simulink model "space_shuttle"  (R2020a)
settings: Solver=ode45  StartTime=0.0  StopTime=8  FixedStep=ts  MaxStep=tpwm/100  RelTol=1e-3
values from neighbouring files (symbols this model uses):
  alphac0 = 0.30    (= 0.3)    [main.m]
  alphac1 = 0.27    [main.m]
  alphanom = 0.3    [main.m]
  E = 0.05    [main.m]
  Kd = 0.75    [main.m]
  Ki = 2.70    (= 2.7)    [main.m]
  Kp = 1.25    [main.m]
  tpwm = 0.02    [main.m]
  ts = 0.1    [main.m]
  tstep = 1    [equarec.m]    (also in main.m; navettecontinue.m)
  u0 = 0    [main.m]
  u1 = 0.05    [main.m]
  x0 = [0;0]    [main.m]    (also in ore.m = x0(:))
undefined symbols (not defined in the file or in its folder): denctf, dendtf, DiscIntNeverNeededParam, numctf, numdtf
libraries: simulink x4
settings Model: Creator=albanfelix  LastModifiedBy=albanfelix

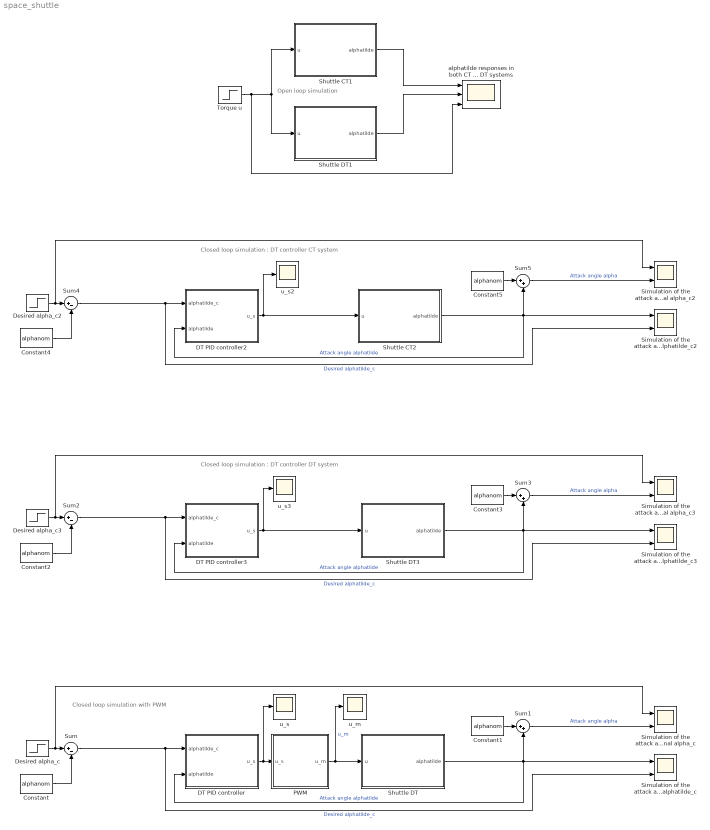
== system space_shuttle ==
  note: Open loop simulation
  note: Closed loop simulation with PWM
  note: Closed loop simulation : DT controller DT system
  note: Closed loop simulation : DT controller CT system
  Constant{,1..5} (6 alike) : Constant  Value=alphanom  SampleTime=ts
  DT PID controller : Subsystem
  DT PID controller2 : Subsystem
  DT PID controller3 : Subsystem
  Desired alpha_c : Step  Time=tstep  Before=alphac0  After=alphac1  SampleTime=ts
  Desired alpha_c2 : Step  Time=tstep  Before=alphac0  After=alphac1  SampleTime=ts
  Desired alpha_c3 : Step  Time=tstep  Before=alphac0  After=alphac1  SampleTime=ts
  PWM : Subsystem
  Shuttle CT1 : Subsystem
  Shuttle CT2 : Subsystem
  Shuttle DT : Subsystem
  Shuttle DT1 : Subsystem
  Shuttle DT3 : Subsystem
  Simulation of the attack angle alpha in function of the desired signal alpha_c : Scope  NumInputPorts=2
  Simulation of the attack angle alpha in function of the desired signal alpha_c2 : Scope  NumInputPorts=2
  Simulation of the attack angle alpha in function of the desired signal alpha_c3 : Scope  NumInputPorts=2
  Simulation of the attack angle alphatilde in function of the desired signal alphatilde_c : Scope  NumInputPorts=2
  Simulation of the attack angle alphatilde in function of the desired signal alphatilde_c2 : Scope  NumInputPorts=2
  Simulation of the attack angle alphatilde in function of the desired signal alphatilde_c3 : Scope  NumInputPorts=2
  Sum : Sum  Inputs=|+-
  Sum1 : Sum  Inputs=|++
  Sum2 : Sum  Inputs=|+-
  Sum3 : Sum  Inputs=|++
  Sum4 : Sum  Inputs=|+-
  Sum5 : Sum  Inputs=|++
  Torque u : Step  Time=tstep  Before=u0  After=u1  SampleTime=ts
  alphatilde responses in both CT and DT systems : Scope  NumInputPorts=3
  u_m : Scope
  u_s : Scope
  u_s2 : Scope
  u_s3 : Scope
  wires:
  Shuttle DT1/1(alphatilde) -> alphatilde responses in both CT and DT systems/2
  Shuttle DT/1(alphatilde) -> Simulation of the attack angle alphatilde in function of the desired signal alphatilde_c/1, DT PID controller/2(alphatilde), Sum1/2  "Attack angle alphatilde"
  DT PID controller/1(u_s) -> u_s/1, PWM/1(u_s)
  PWM/1(u_m) -> Shuttle DT/1(u), u_m/1  "u_m"
  Shuttle CT1/1(alphatilde) -> alphatilde responses in both CT and DT systems/1
  Sum/1 -> Simulation of the attack angle alphatilde in function of the desired signal alphatilde_c/2, DT PID controller/1(alphatilde_c)  "Desired alphatilde_c"
  Desired alpha_c/1 -> Simulation of the attack angle alpha in function of the desired signal alpha_c/1, Sum/1
  Constant/1 -> Sum/2
  Constant1/1 -> Sum1/1
  Sum1/1 -> Simulation of the attack angle alpha in function of the desired signal alpha_c/2  "Attack angle alpha"
  DT PID controller3/1(u_s) -> u_s3/1, Shuttle DT3/1(u)
  Sum3/1 -> Simulation of the attack angle alpha in function of the desired signal alpha_c3/2  "Attack angle alpha"
  Shuttle DT3/1(alphatilde) -> Simulation of the attack angle alphatilde in function of the desired signal alphatilde_c3/1, DT PID controller3/2(alphatilde), Sum3/2  "Attack angle alphatilde"
  Sum2/1 -> Simulation of the attack angle alphatilde in function of the desired signal alphatilde_c3/2, DT PID controller3/1(alphatilde_c)  "Desired alphatilde_c"
  Desired alpha_c3/1 -> Simulation of the attack angle alpha in function of the desired signal alpha_c3/1, Sum2/1
  Constant2/1 -> Sum2/2
  Constant3/1 -> Sum3/1
  Sum5/1 -> Simulation of the attack angle alpha in function of the desired signal alpha_c2/2  "Attack angle alpha"
  Constant5/1 -> Sum5/1
  Constant4/1 -> Sum4/2
  Desired alpha_c2/1 -> Simulation of the attack angle alpha in function of the desired signal alpha_c2/1, Sum4/1
  DT PID controller2/1(u_s) -> Shuttle CT2/1(u), u_s2/1
  Shuttle CT2/1(alphatilde) -> Simulation of the attack angle alphatilde in function of the desired signal alphatilde_c2/1, DT PID controller2/2(alphatilde), Sum5/2  "Attack angle alphatilde"
  Sum4/1 -> Simulation of the attack angle alphatilde in function of the desired signal alphatilde_c2/2, DT PID controller2/1(alphatilde_c)  "Desired alphatilde_c"
  Torque u/1 -> alphatilde responses in both CT and DT systems/3, Shuttle CT1/1(u), Shuttle DT1/1(u)

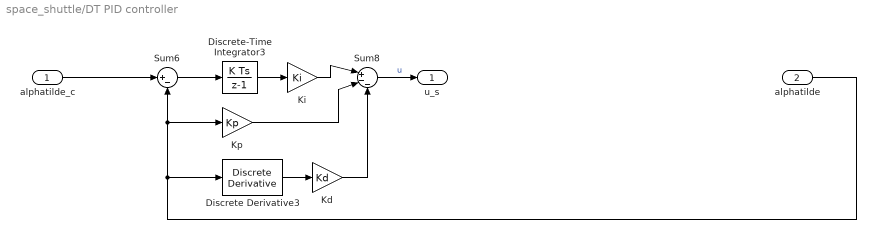
== system space_shuttle/DT PID controller ==
  alphatilde_c : Inport
  alphatilde : Inport  Port=2
  Discrete Derivative3 : simulink/Discrete/Discrete Derivative  gainval=1.0  ICPrevScaledInput=0.0  OutMin=[]  OutMax=[]  OutDataType=fixdt(1, 16)  OutScaling=2^-10  DoSatur=off
  Discrete-Time Integrator3 : DiscreteIntegrator  SampleTime=ts  ICPrevOutput=DiscIntNeverNeededParam  ICPrevScaledInput=DiscIntNeverNeededParam
  Kd : Gain  Gain=Kd
  Ki : Gain  Gain=Ki
  Kp : Gain  Gain=Kp
  Sum6 : Sum  Inputs=|+-
  Sum8 : Sum  Inputs=|+--
  u_s : Outport
  wires:
  Ki/1 -> Sum8/1
  Sum8/1 -> u_s/1  "u"
  Sum6/1 -> Discrete-Time Integrator3/1
  Discrete Derivative3/1 -> Kd/1
  alphatilde_c/1 -> Sum6/1
  Kp/1 -> Sum8/2
  Kd/1 -> Sum8/3
  Discrete-Time Integrator3/1 -> Ki/1
  alphatilde/1 -> Kp/1, Sum6/2, Discrete Derivative3/1

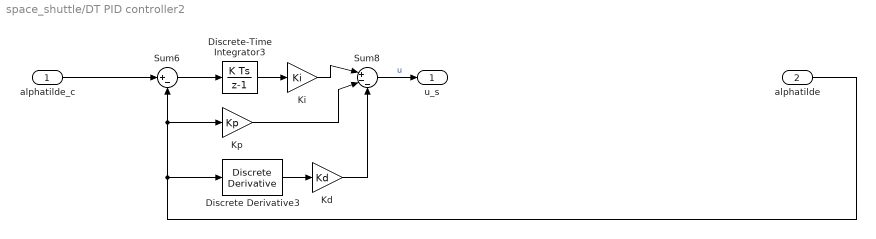
== system space_shuttle/DT PID controller2 ==
  alphatilde_c : Inport
  alphatilde : Inport  Port=2
  Discrete Derivative3 : simulink/Discrete/Discrete Derivative  gainval=1.0  ICPrevScaledInput=0.0  OutMin=[]  OutMax=[]  OutDataType=fixdt(1, 16)  OutScaling=2^-10  DoSatur=off
  Discrete-Time Integrator3 : DiscreteIntegrator  SampleTime=ts  ICPrevOutput=DiscIntNeverNeededParam  ICPrevScaledInput=DiscIntNeverNeededParam
  Kd : Gain  Gain=Kd
  Ki : Gain  Gain=Ki
  Kp : Gain  Gain=Kp
  Sum6 : Sum  Inputs=|+-
  Sum8 : Sum  Inputs=|+--
  u_s : Outport
  wires:
  Ki/1 -> Sum8/1
  Sum8/1 -> u_s/1  "u"
  Sum6/1 -> Discrete-Time Integrator3/1
  Discrete Derivative3/1 -> Kd/1
  alphatilde_c/1 -> Sum6/1
  Kp/1 -> Sum8/2
  Kd/1 -> Sum8/3
  Discrete-Time Integrator3/1 -> Ki/1
  alphatilde/1 -> Kp/1, Sum6/2, Discrete Derivative3/1

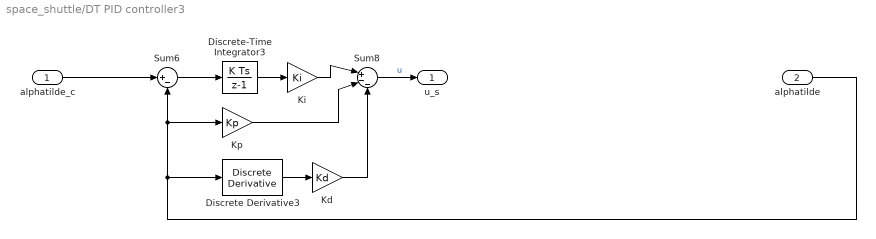
== system space_shuttle/DT PID controller3 ==
  alphatilde_c : Inport
  alphatilde : Inport  Port=2
  Discrete Derivative3 : simulink/Discrete/Discrete Derivative  gainval=1.0  ICPrevScaledInput=0.0  OutMin=[]  OutMax=[]  OutDataType=fixdt(1, 16)  OutScaling=2^-10  DoSatur=off
  Discrete-Time Integrator3 : DiscreteIntegrator  SampleTime=ts  ICPrevOutput=DiscIntNeverNeededParam  ICPrevScaledInput=DiscIntNeverNeededParam
  Kd : Gain  Gain=Kd
  Ki : Gain  Gain=Ki
  Kp : Gain  Gain=Kp
  Sum6 : Sum  Inputs=|+-
  Sum8 : Sum  Inputs=|+--
  u_s : Outport
  wires:
  Ki/1 -> Sum8/1
  Sum8/1 -> u_s/1  "u"
  Sum6/1 -> Discrete-Time Integrator3/1
  Discrete Derivative3/1 -> Kd/1
  alphatilde_c/1 -> Sum6/1
  Kp/1 -> Sum8/2
  Kd/1 -> Sum8/3
  Discrete-Time Integrator3/1 -> Ki/1
  alphatilde/1 -> Kp/1, Sum6/2, Discrete Derivative3/1

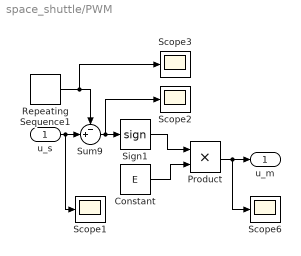
== system space_shuttle/PWM ==
  u_s : Inport
  Constant : Constant  Value=E  SampleTime=ts
  Product : Product
  Repeating Sequence1 : simulink/Sources/Repeating Sequence  rep_seq_t=[0,tpwm/2,tpwm]  rep_seq_y=[-E,E,-E]
  Scope{1..3,6} (4 alike) : Scope
  Sign1 : Signum
  Sum9 : Sum  Inputs=-+|
  u_m : Outport
  wires:
  u_s/1 -> Scope1/1, Sum9/2
  Sum9/1 -> Scope2/1, Sign1/1
  Repeating Sequence1/1 -> Scope3/1, Sum9/1
  Product/1 -> Scope6/1, u_m/1
  Constant/1 -> Product/2
  Sign1/1 -> Product/1

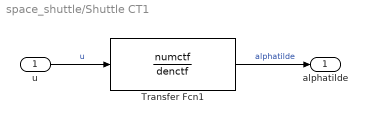
== system space_shuttle/Shuttle CT1 ==
  u : Inport
  Transfer Fcn1 : TransferFcn  Numerator=numctf  Denominator=denctf
  alphatilde : Outport
  wires:
  u/1 -> Transfer Fcn1/1  "u"
  Transfer Fcn1/1 -> alphatilde/1  "alphatilde"

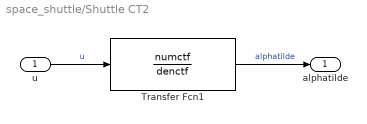
== system space_shuttle/Shuttle CT2 ==
  u : Inport
  Transfer Fcn1 : TransferFcn  Numerator=numctf  Denominator=denctf
  alphatilde : Outport
  wires:
  u/1 -> Transfer Fcn1/1  "u"
  Transfer Fcn1/1 -> alphatilde/1  "alphatilde"

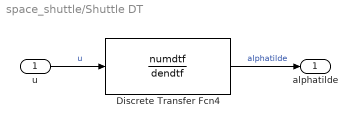
== system space_shuttle/Shuttle DT ==
  u : Inport
  Discrete Transfer Fcn4 : DiscreteTransferFcn  Numerator=numdtf  Denominator=dendtf  InitialStates=x0  SampleTime=ts
  alphatilde : Outport
  wires:
  u/1 -> Discrete Transfer Fcn4/1  "u"
  Discrete Transfer Fcn4/1 -> alphatilde/1  "alphatilde"

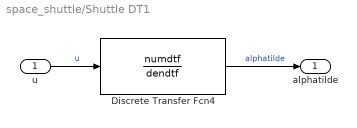
== system space_shuttle/Shuttle DT1 ==
  u : Inport
  Discrete Transfer Fcn4 : DiscreteTransferFcn  Numerator=numdtf  Denominator=dendtf  InitialStates=x0  SampleTime=ts
  alphatilde : Outport
  wires:
  u/1 -> Discrete Transfer Fcn4/1  "u"
  Discrete Transfer Fcn4/1 -> alphatilde/1  "alphatilde"

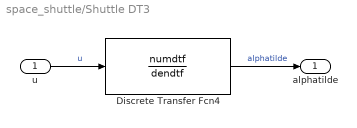
== system space_shuttle/Shuttle DT3 ==
  u : Inport
  Discrete Transfer Fcn4 : DiscreteTransferFcn  Numerator=numdtf  Denominator=dendtf  InitialStates=x0  SampleTime=ts
  alphatilde : Outport
  wires:
  u/1 -> Discrete Transfer Fcn4/1  "u"
  Discrete Transfer Fcn4/1 -> alphatilde/1  "alphatilde"
